simulink model "referee"  (R2018a)
settings: Solver=VariableStepAuto  StartTime=0.0  StopTime=20  FixedStep=0.01  RelTol=1e-3
libraries: simulink x16, instrumentlib x2
settings Model: EnablePacing=on  Creator=U500304  LastModifiedBy=Rafael
settings SolverCC: ZeroCrossAlgorithm=Adaptive
settings DataIOCC: SaveOutput=off  SaveTime=off
settings DebuggingCC: MaxConsecutiveZCsMsg=none

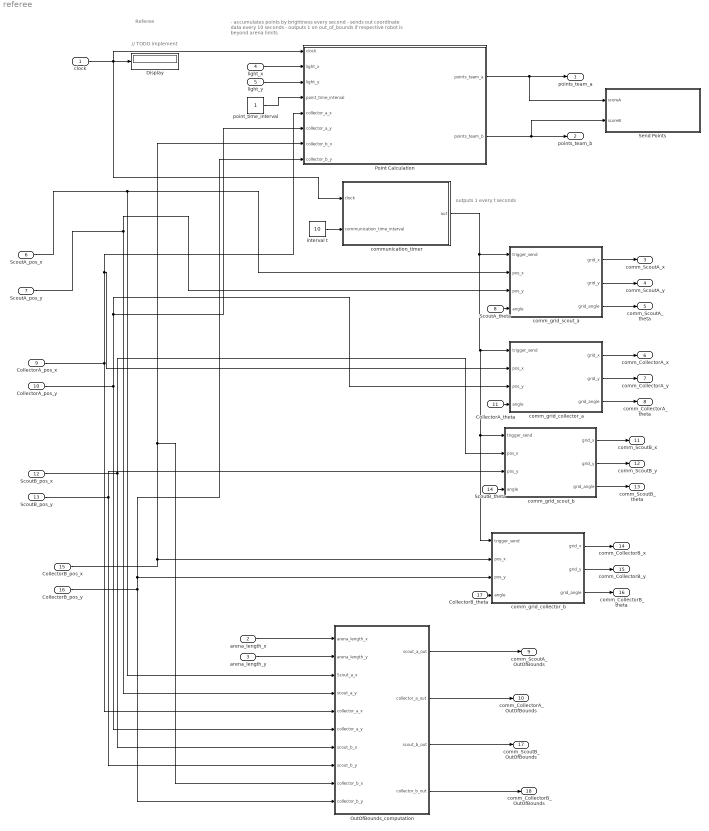
== system referee ==
  note: - accumulates points by brightness every second
      | - sends out coordinate data every 10 seconds
      | - outputs 1 on out_of_bounds if respective robot is beyond arena limits
  note: outputs 1 every t seconds
  note: // TODO implement
  note: Referee
  clock : Inport  OutDataTypeStr=double  PortDimensions=1  SampleTime=0
  arena_length_x : Inport  Port=2
  arena_length_y : Inport  Port=3
  light_x : Inport  Port=4
  light_y : Inport  Port=5
  ScoutA_pos_x : Inport  Port=6
  ScoutA_pos_y : Inport  Port=7
  ScoutA_theta : Inport  Port=8
  CollectorA_pos_x : Inport  Port=9
  CollectorA_pos_y : Inport  Port=10
  CollectorA_theta : Inport  Port=11
  ScoutB_pos_x : Inport  Port=12
  ScoutB_pos_y : Inport  Port=13
  ScoutB_theta : Inport  Port=14
  CollectorB_pos_x : Inport  Port=15
  CollectorB_pos_y : Inport  Port=16
  CollectorB_theta : Inport  Port=17
  Display : Display
  OutOfBounds_computation : Subsystem
  Point Calculation : Subsystem
  Send Points : Subsystem
  comm_grid_collector_a : Subsystem
  comm_grid_collector_b : Subsystem
  "comm_grid_scout_a " : Subsystem
  comm_grid_scout_b : Subsystem
  communication_timer : Subsystem
  interval t : Constant  Value=10
  point_time_interval : Constant
  points_team_a : Outport
  points_team_b : Outport  Port=2
  comm_ScoutA_x : Outport  Port=3
  comm_ScoutA_y : Outport  Port=4
  comm_ScoutA_theta : Outport  Port=5
  comm_CollectorA_x : Outport  Port=6
  comm_CollectorA_y : Outport  Port=7
  comm_CollectorA_theta : Outport  Port=8
  comm_ScoutA_OutOfBounds : Outport  Port=9
  comm_CollectorA_OutOfBounds : Outport  Port=10
  comm_ScoutB_x : Outport  Port=11
  comm_ScoutB_y : Outport  Port=12
  comm_ScoutB_theta : Outport  Port=13
  comm_CollectorB_x : Outport  Port=14
  comm_CollectorB_y : Outport  Port=15
  comm_CollectorB_theta : Outport  Port=16
  comm_ScoutB_OutOfBounds : Outport  Port=17
  comm_CollectorB_OutOfBounds : Outport  Port=18
  wires:
  arena_length_x/1 -> OutOfBounds_computation/1(arena_length_x)
  arena_length_y/1 -> OutOfBounds_computation/2(arena_length_y)
  ScoutA_pos_x/1 -> "comm_grid_scout_a "/2(pos_x), OutOfBounds_computation/3(Scout_a_x)
  ScoutA_pos_y/1 -> "comm_grid_scout_a "/3(pos_y), OutOfBounds_computation/4(scout_a_y)
  CollectorA_pos_x/1 -> comm_grid_collector_a/2(pos_x), Point Calculation/5(collector_a_x), OutOfBounds_computation/5(collector_a_x)
  CollectorA_pos_y/1 -> comm_grid_collector_a/3(pos_y), Point Calculation/6(collector_a_y), OutOfBounds_computation/6(collector_a_y)
  ScoutB_pos_x/1 -> comm_grid_scout_b/2(pos_x), OutOfBounds_computation/7(scout_b_x)
  ScoutB_pos_y/1 -> comm_grid_scout_b/3(pos_y), OutOfBounds_computation/8(scout_b_y)
  CollectorB_pos_x/1 -> Point Calculation/7(collector_b_x), OutOfBounds_computation/9(collector_b_x), comm_grid_collector_b/2(pos_x)
  CollectorB_pos_y/1 -> Point Calculation/8(collector_b_y), comm_grid_collector_b/3(pos_y), OutOfBounds_computation/10(collector_b_y)
  OutOfBounds_computation/1(scout_a_out) -> comm_ScoutA_OutOfBounds/1
  OutOfBounds_computation/2(collector_a_out) -> comm_CollectorA_OutOfBounds/1
  OutOfBounds_computation/3(scout_b_out) -> comm_ScoutB_OutOfBounds/1
  OutOfBounds_computation/4(collector_b_out) -> comm_CollectorB_OutOfBounds/1
  light_x/1 -> Point Calculation/2(light_x)
  light_y/1 -> Point Calculation/3(light_y)
  point_time_interval/1 -> Point Calculation/4(point_time_interval)
  Point Calculation/1(points_team_a) -> Send Points/1(scoreA), points_team_a/1
  Point Calculation/2(points_team_b) -> points_team_b/1, Send Points/2(scoreB)
  clock/1 -> communication_timer/1(clock), Point Calculation/1("clock "), Display/1
  interval t/1 -> communication_timer/2(communication_time_interval)
  communication_timer/1(out) -> comm_grid_collector_b/1(trigger_send), comm_grid_scout_b/1(trigger_send), comm_grid_collector_a/1(trigger_send), "comm_grid_scout_a "/1(trigger_send)
  ScoutA_theta/1 -> "comm_grid_scout_a "/4(angle)
  "comm_grid_scout_a "/1(grid_x) -> comm_ScoutA_x/1
  "comm_grid_scout_a "/2(grid_y) -> comm_ScoutA_y/1
  "comm_grid_scout_a "/3(grid_angle) -> comm_ScoutA_theta/1
  CollectorA_theta/1 -> comm_grid_collector_a/4(angle)
  comm_grid_collector_a/1(grid_x) -> comm_CollectorA_x/1
  comm_grid_collector_a/2(grid_y) -> comm_CollectorA_y/1
  comm_grid_collector_a/3(grid_angle) -> comm_CollectorA_theta/1
  ScoutB_theta/1 -> comm_grid_scout_b/4(angle)
  comm_grid_scout_b/1(grid_x) -> comm_ScoutB_x/1
  comm_grid_scout_b/2(grid_y) -> comm_ScoutB_y/1
  comm_grid_scout_b/3(grid_angle) -> comm_ScoutB_theta/1
  CollectorB_theta/1 -> comm_grid_collector_b/4(angle)
  comm_grid_collector_b/1(grid_x) -> comm_CollectorB_x/1
  comm_grid_collector_b/2(grid_y) -> comm_CollectorB_y/1
  comm_grid_collector_b/3(grid_angle) -> comm_CollectorB_theta/1

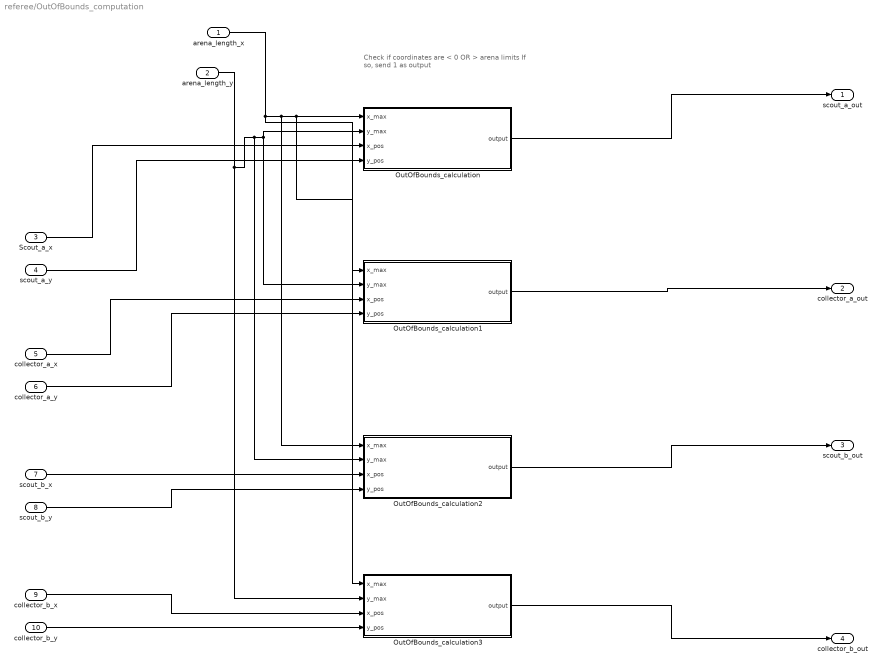
== system referee/OutOfBounds_computation ==
  note: Check if coordinates are < 0 OR > arena limits
      | If so, send 1 as output
  arena_length_x : Inport
  arena_length_y : Inport  Port=2
  Scout_a_x : Inport  Port=3
  scout_a_y : Inport  Port=4
  collector_a_x : Inport  Port=5
  collector_a_y : Inport  Port=6
  scout_b_x : Inport  Port=7
  scout_b_y : Inport  Port=8
  collector_b_x : Inport  Port=9
  collector_b_y : Inport  Port=10
  OutOfBounds_calculation : Subsystem
  OutOfBounds_calculation1 : Subsystem
  OutOfBounds_calculation2 : Subsystem
  OutOfBounds_calculation3 : Subsystem
  scout_a_out : Outport
  collector_a_out : Outport  Port=2
  scout_b_out : Outport  Port=3
  collector_b_out : Outport  Port=4
  wires:
  OutOfBounds_calculation/1(output) -> scout_a_out/1
  arena_length_x/1 -> OutOfBounds_calculation3/1(x_max), OutOfBounds_calculation2/1(x_max), OutOfBounds_calculation1/1(x_max), OutOfBounds_calculation/1(x_max)
  arena_length_y/1 -> OutOfBounds_calculation3/2(y_max), OutOfBounds_calculation2/2(y_max), OutOfBounds_calculation/2(y_max), OutOfBounds_calculation1/2(y_max)
  collector_b_y/1 -> OutOfBounds_calculation3/4(y_pos)
  OutOfBounds_calculation1/1(output) -> collector_a_out/1
  collector_b_x/1 -> OutOfBounds_calculation3/3(x_pos)
  collector_a_y/1 -> OutOfBounds_calculation1/4(y_pos)
  scout_b_x/1 -> OutOfBounds_calculation2/3(x_pos)
  OutOfBounds_calculation2/1(output) -> scout_b_out/1
  Scout_a_x/1 -> OutOfBounds_calculation/3(x_pos)
  scout_a_y/1 -> OutOfBounds_calculation/4(y_pos)
  OutOfBounds_calculation3/1(output) -> collector_b_out/1
  scout_b_y/1 -> OutOfBounds_calculation2/4(y_pos)
  collector_a_x/1 -> OutOfBounds_calculation1/3(x_pos)

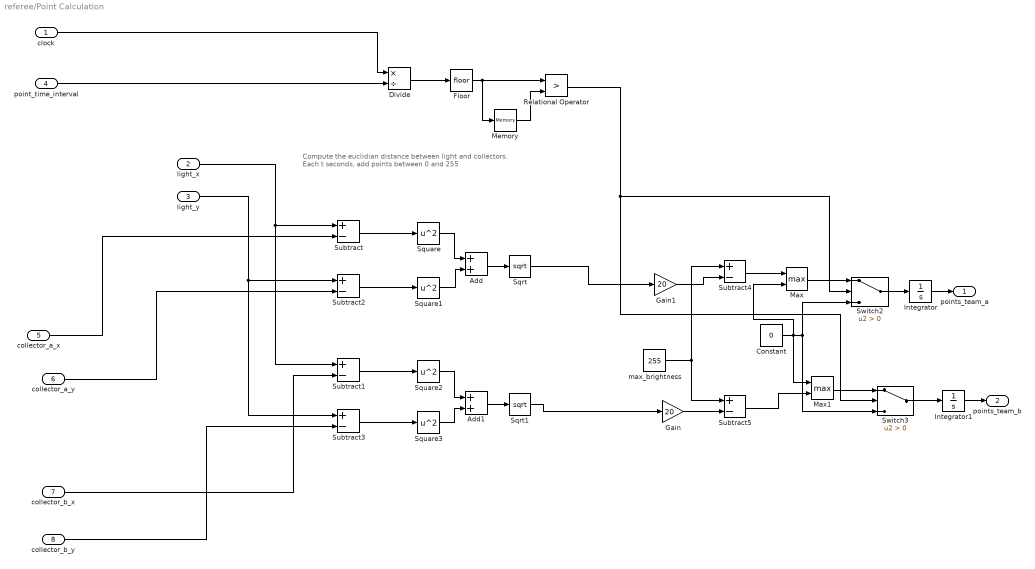
== system referee/Point Calculation ==
  note: Compute the euclidian distance between light and collectors.
      | Each t seconds, add points between 0 and 255
  "clock " : Inport
  light_x : Inport  Port=2
  light_y : Inport  Port=3
  point_time_interval : Inport  Port=4
  collector_a_x : Inport  Port=5
  collector_a_y : Inport  Port=6
  collector_b_x : Inport  Port=7
  collector_b_y : Inport  Port=8
  Add : Sum
  Add1 : Sum
  Constant : Constant  Value=0
  Divide : Product  Inputs=*/
  Floor : Rounding
  Gain : Gain  Gain=20
  Gain1 : Gain  Gain=20
  Integrator : Integrator
  Integrator1 : Integrator
  Max : MinMax  Function=max  Inputs=2
  Max1 : MinMax  Function=max  Inputs=2
  Memory : Memory
  Relational Operator : RelationalOperator  Operator=>  OutDataTypeStr=boolean  RndMeth=Simplest
  Sqrt : Sqrt  SaturateOnIntegerOverflow=on
  Sqrt1 : Sqrt  SaturateOnIntegerOverflow=on
  Square{,1..3} (4 alike) : Math  Operator=square  SaturateOnIntegerOverflow=on
  Subtract{,1..5} (6 alike) : Sum  Inputs=+-
  Switch2 : Switch  Criteria=u2 > Threshold
  Switch3 : Switch  Criteria=u2 > Threshold
  max_brightness : Constant  Value=255
  points_team_a : Outport
  points_team_b : Outport  Port=2
  wires:
  Divide/1 -> Floor/1
  light_y/1 -> Subtract3/1, Subtract2/1
  Memory/1 -> Relational Operator/2
  light_x/1 -> Subtract1/1, Subtract/1
  Square/1 -> Add/1
  Floor/1 -> Relational Operator/1, Memory/1
  collector_b_y/1 -> Subtract3/2
  Add/1 -> Sqrt/1
  Constant/1 -> Max1/1, Max/2, Switch3/3, Switch2/3
  Relational Operator/1 -> Switch3/2, Switch2/2
  point_time_interval/1 -> Divide/2
  collector_a_x/1 -> Subtract/2
  Square3/1 -> Add1/2
  Subtract2/1 -> Square1/1
  Subtract/1 -> Square/1
  Subtract1/1 -> Square2/1
  Add1/1 -> Sqrt1/1
  Square2/1 -> Add1/1
  Subtract3/1 -> Square3/1
  Square1/1 -> Add/2
  collector_a_y/1 -> Subtract2/2
  collector_b_x/1 -> Subtract1/2
  "clock "/1 -> Divide/1
  max_brightness/1 -> Subtract5/1, Subtract4/1
  Sqrt/1 -> Gain1/1
  Gain1/1 -> Subtract4/2
  Subtract4/1 -> Max/1
  Sqrt1/1 -> Gain/1
  Gain/1 -> Subtract5/2
  Subtract5/1 -> Max1/2
  Max/1 -> Switch2/1
  Max1/1 -> Switch3/1
  Integrator/1 -> points_team_a/1
  Integrator1/1 -> points_team_b/1
  Switch3/1 -> Integrator1/1
  Switch2/1 -> Integrator/1

== system referee/Send Points ==
  scoreA : Inport
  scoreB : Inport  Port=2
  Rate Transition5 : RateTransition  OutPortSampleTime=0.1
  Rate Transition6 : RateTransition  OutPortSampleTime=0.1
  tcp_send_scoreA : instrumentlib/TCP//IP Send  Host=localhost  Port=50015  EnableBlockingMode=on  Timeout=1  ByteOrder=LittleEndian  TransferDelay=on
      settings: SourceProductName=Instrument Control Toolbox
  tcp_send_scoreB : instrumentlib/TCP//IP Send  Host=localhost  Port=50016  EnableBlockingMode=on  Timeout=1  ByteOrder=LittleEndian  TransferDelay=on
      settings: SourceProductName=Instrument Control Toolbox
  wires:
  scoreA/1 -> Rate Transition5/1
  scoreB/1 -> Rate Transition6/1
  Rate Transition5/1 -> tcp_send_scoreA/1
  Rate Transition6/1 -> tcp_send_scoreB/1

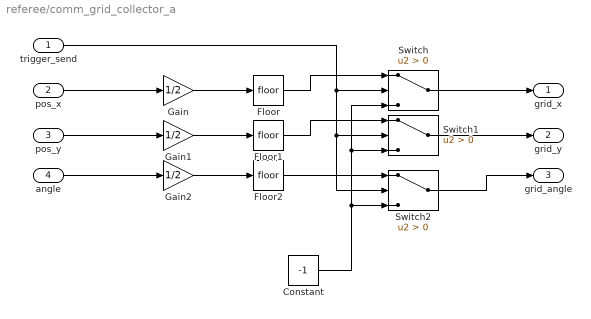
== system referee/comm_grid_collector_a ==
  trigger_send : Inport
  pos_x : Inport  Port=2
  pos_y : Inport  Port=3
  angle : Inport  Port=4
  Constant : Constant  Value=-1
  Floor : Rounding
  Floor1 : Rounding
  Floor2 : Rounding
  Gain : Gain  Gain=1/2
  Gain1 : Gain  Gain=1/2
  Gain2 : Gain  Gain=1/2
  Switch : Switch  Criteria=u2 > Threshold
  Switch1 : Switch  Criteria=u2 > Threshold
  Switch2 : Switch  Criteria=u2 > Threshold
  grid_x : Outport
  grid_y : Outport  Port=2
  grid_angle : Outport  Port=3
  wires:
  Switch2/1 -> grid_angle/1
  Floor/1 -> Switch/1
  Switch/1 -> grid_x/1
  Switch1/1 -> grid_y/1
  angle/1 -> Gain2/1
  Gain2/1 -> Floor2/1
  Floor1/1 -> Switch1/1
  pos_x/1 -> Gain/1
  Gain/1 -> Floor/1
  Gain1/1 -> Floor1/1
  pos_y/1 -> Gain1/1
  trigger_send/1 -> Switch/2, Switch2/2, Switch1/2
  Constant/1 -> Switch1/3, Switch/3, Switch2/3
  Floor2/1 -> Switch2/1

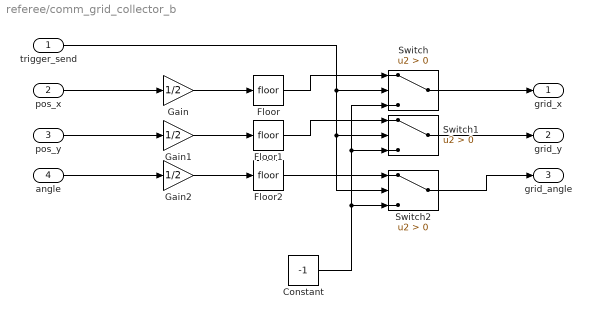
== system referee/comm_grid_collector_b ==
  trigger_send : Inport
  pos_x : Inport  Port=2
  pos_y : Inport  Port=3
  angle : Inport  Port=4
  Constant : Constant  Value=-1
  Floor : Rounding
  Floor1 : Rounding
  Floor2 : Rounding
  Gain : Gain  Gain=1/2
  Gain1 : Gain  Gain=1/2
  Gain2 : Gain  Gain=1/2
  Switch : Switch  Criteria=u2 > Threshold
  Switch1 : Switch  Criteria=u2 > Threshold
  Switch2 : Switch  Criteria=u2 > Threshold
  grid_x : Outport
  grid_y : Outport  Port=2
  grid_angle : Outport  Port=3
  wires:
  Floor2/1 -> Switch2/1
  Constant/1 -> Switch2/3, Switch/3, Switch1/3
  trigger_send/1 -> Switch1/2, Switch2/2, Switch/2
  pos_y/1 -> Gain1/1
  Gain1/1 -> Floor1/1
  Gain/1 -> Floor/1
  pos_x/1 -> Gain/1
  Floor1/1 -> Switch1/1
  Gain2/1 -> Floor2/1
  angle/1 -> Gain2/1
  Switch1/1 -> grid_y/1
  Switch/1 -> grid_x/1
  Floor/1 -> Switch/1
  Switch2/1 -> grid_angle/1

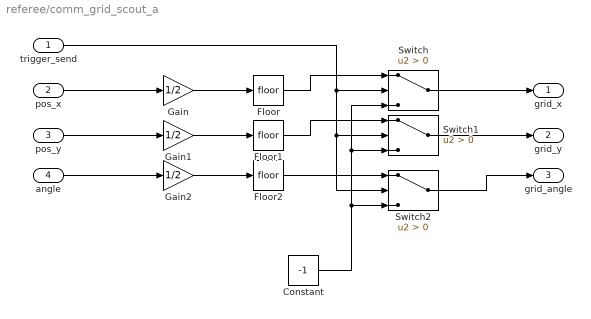
== system referee/comm_grid_scout_a  ==
  trigger_send : Inport
  pos_x : Inport  Port=2
  pos_y : Inport  Port=3
  angle : Inport  Port=4
  Constant : Constant  Value=-1
  Floor : Rounding
  Floor1 : Rounding
  Floor2 : Rounding
  Gain : Gain  Gain=1/2
  Gain1 : Gain  Gain=1/2
  Gain2 : Gain  Gain=1/2
  Switch : Switch  Criteria=u2 > Threshold
  Switch1 : Switch  Criteria=u2 > Threshold
  Switch2 : Switch  Criteria=u2 > Threshold
  grid_x : Outport
  grid_y : Outport  Port=2
  grid_angle : Outport  Port=3
  wires:
  Floor2/1 -> Switch2/1
  Constant/1 -> Switch2/3, Switch/3, Switch1/3
  trigger_send/1 -> Switch1/2, Switch2/2, Switch/2
  pos_y/1 -> Gain1/1
  Gain1/1 -> Floor1/1
  Gain/1 -> Floor/1
  pos_x/1 -> Gain/1
  Floor1/1 -> Switch1/1
  Gain2/1 -> Floor2/1
  angle/1 -> Gain2/1
  Switch1/1 -> grid_y/1
  Switch/1 -> grid_x/1
  Floor/1 -> Switch/1
  Switch2/1 -> grid_angle/1

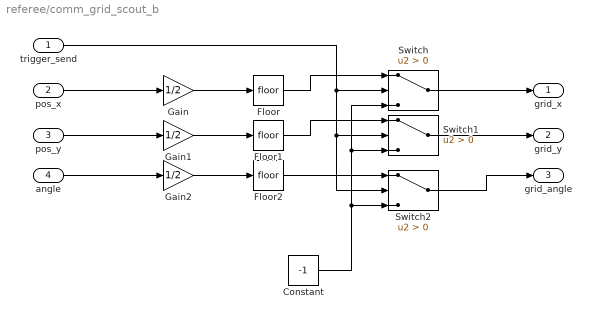
== system referee/comm_grid_scout_b ==
  trigger_send : Inport
  pos_x : Inport  Port=2
  pos_y : Inport  Port=3
  angle : Inport  Port=4
  Constant : Constant  Value=-1
  Floor : Rounding
  Floor1 : Rounding
  Floor2 : Rounding
  Gain : Gain  Gain=1/2
  Gain1 : Gain  Gain=1/2
  Gain2 : Gain  Gain=1/2
  Switch : Switch  Criteria=u2 > Threshold
  Switch1 : Switch  Criteria=u2 > Threshold
  Switch2 : Switch  Criteria=u2 > Threshold
  grid_x : Outport
  grid_y : Outport  Port=2
  grid_angle : Outport  Port=3
  wires:
  Switch2/1 -> grid_angle/1
  Floor/1 -> Switch/1
  Switch/1 -> grid_x/1
  Switch1/1 -> grid_y/1
  angle/1 -> Gain2/1
  Gain2/1 -> Floor2/1
  Floor1/1 -> Switch1/1
  pos_x/1 -> Gain/1
  Gain/1 -> Floor/1
  Gain1/1 -> Floor1/1
  pos_y/1 -> Gain1/1
  trigger_send/1 -> Switch/2, Switch2/2, Switch1/2
  Constant/1 -> Switch1/3, Switch/3, Switch2/3
  Floor2/1 -> Switch2/1

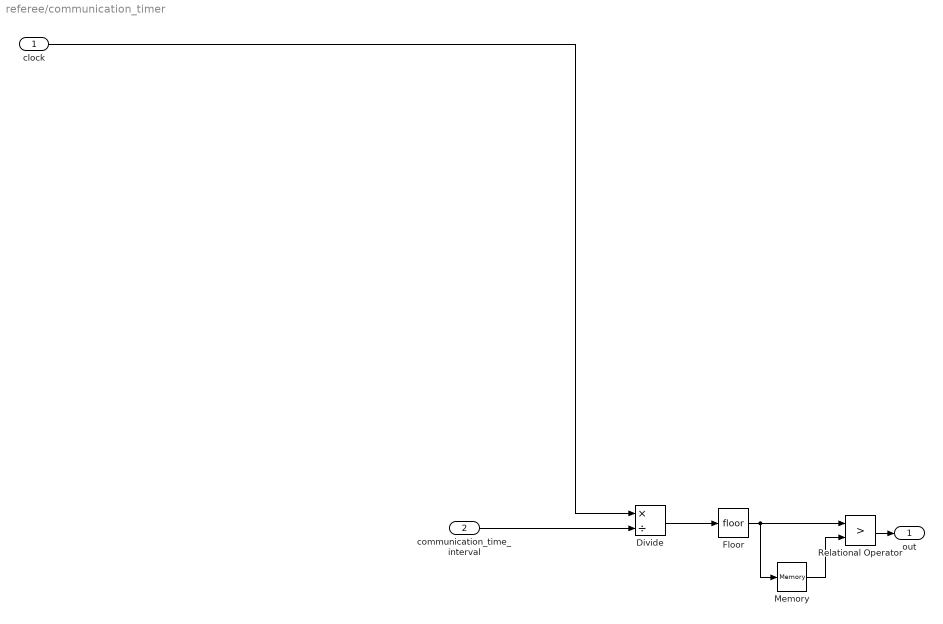
== system referee/communication_timer ==
  clock : Inport
  communication_time_interval : Inport  Port=2
  Divide : Product  Inputs=*/
  Floor : Rounding
  Memory : Memory
  Relational Operator : RelationalOperator  Operator=>  OutDataTypeStr=boolean  RndMeth=Simplest
  out : Outport
  wires:
  Divide/1 -> Floor/1
  Memory/1 -> Relational Operator/2
  Floor/1 -> Relational Operator/1, Memory/1
  communication_time_interval/1 -> Divide/2
  clock/1 -> Divide/1
  Relational Operator/1 -> out/1

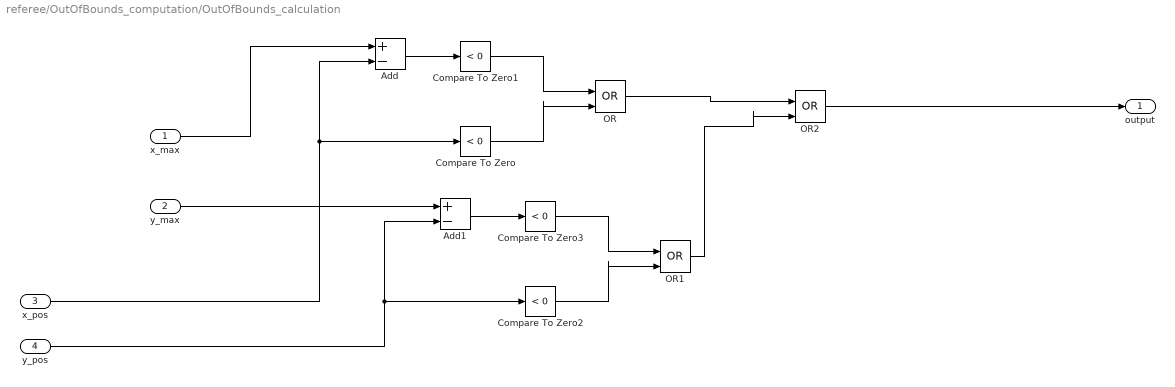
== system referee/OutOfBounds_computation/OutOfBounds_calculation ==
  x_max : Inport
  y_max : Inport  Port=2
  x_pos : Inport  Port=3
  y_pos : Inport  Port=4
  Add : Sum  Inputs=+-
  Add1 : Sum  Inputs=+-
  Compare To Zero{,1..3} (4 alike) : simulink/Logic and Bit Operations/Compare To Zero  relop=<  OutDataTypeStr=boolean
  OR : Logic  Operator=OR  IconShape=distinctive  AllPortsSameDT=off  OutDataTypeStr=boolean
  OR1 : Logic  Operator=OR  IconShape=distinctive  AllPortsSameDT=off  OutDataTypeStr=boolean
  OR2 : Logic  Operator=OR  IconShape=distinctive  AllPortsSameDT=off  OutDataTypeStr=boolean
  output : Outport
  wires:
  Add1/1 -> Compare To Zero3/1
  Compare To Zero3/1 -> OR1/1
  x_pos/1 -> Add/2, Compare To Zero/1
  x_max/1 -> Add/1
  OR/1 -> OR2/1
  y_pos/1 -> Add1/2, Compare To Zero2/1
  Compare To Zero2/1 -> OR1/2
  Compare To Zero/1 -> OR/2
  OR1/1 -> OR2/2
  Add/1 -> Compare To Zero1/1
  Compare To Zero1/1 -> OR/1
  y_max/1 -> Add1/1
  OR2/1 -> output/1

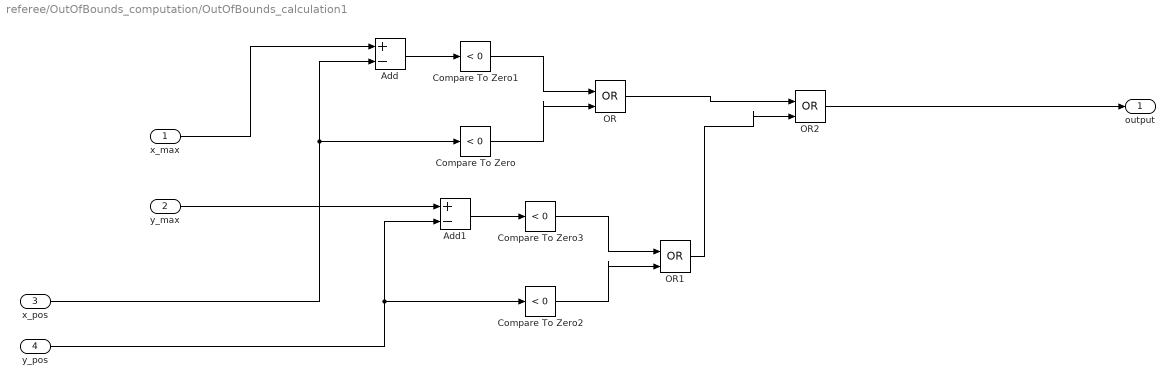
== system referee/OutOfBounds_computation/OutOfBounds_calculation1 ==
  x_max : Inport
  y_max : Inport  Port=2
  x_pos : Inport  Port=3
  y_pos : Inport  Port=4
  Add : Sum  Inputs=+-
  Add1 : Sum  Inputs=+-
  Compare To Zero{,1..3} (4 alike) : simulink/Logic and Bit Operations/Compare To Zero  relop=<  OutDataTypeStr=boolean
  OR : Logic  Operator=OR  IconShape=distinctive  AllPortsSameDT=off  OutDataTypeStr=boolean
  OR1 : Logic  Operator=OR  IconShape=distinctive  AllPortsSameDT=off  OutDataTypeStr=boolean
  OR2 : Logic  Operator=OR  IconShape=distinctive  AllPortsSameDT=off  OutDataTypeStr=boolean
  output : Outport
  wires:
  OR2/1 -> output/1
  y_max/1 -> Add1/1
  Compare To Zero1/1 -> OR/1
  Add/1 -> Compare To Zero1/1
  OR1/1 -> OR2/2
  Compare To Zero/1 -> OR/2
  Compare To Zero2/1 -> OR1/2
  y_pos/1 -> Compare To Zero2/1, Add1/2
  OR/1 -> OR2/1
  x_max/1 -> Add/1
  x_pos/1 -> Compare To Zero/1, Add/2
  Compare To Zero3/1 -> OR1/1
  Add1/1 -> Compare To Zero3/1

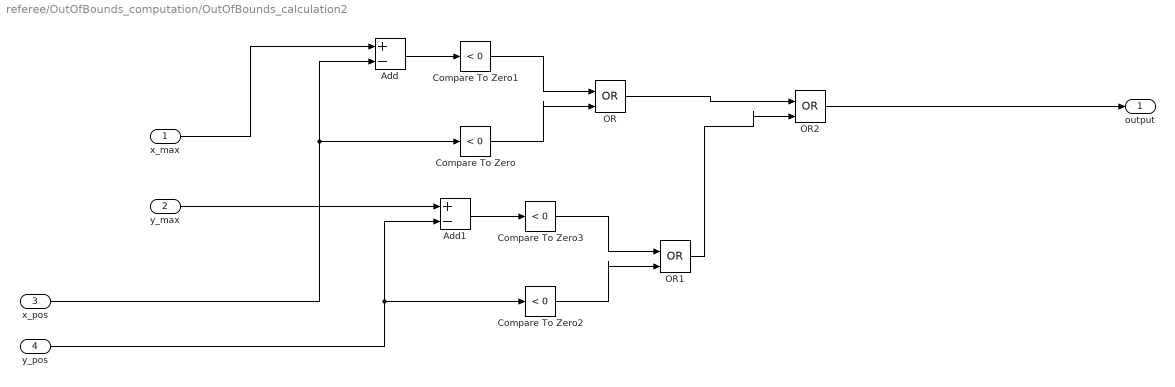
== system referee/OutOfBounds_computation/OutOfBounds_calculation2 ==
  x_max : Inport
  y_max : Inport  Port=2
  x_pos : Inport  Port=3
  y_pos : Inport  Port=4
  Add : Sum  Inputs=+-
  Add1 : Sum  Inputs=+-
  Compare To Zero{,1..3} (4 alike) : simulink/Logic and Bit Operations/Compare To Zero  relop=<  OutDataTypeStr=boolean
  OR : Logic  Operator=OR  IconShape=distinctive  AllPortsSameDT=off  OutDataTypeStr=boolean
  OR1 : Logic  Operator=OR  IconShape=distinctive  AllPortsSameDT=off  OutDataTypeStr=boolean
  OR2 : Logic  Operator=OR  IconShape=distinctive  AllPortsSameDT=off  OutDataTypeStr=boolean
  output : Outport
  wires:
  Add1/1 -> Compare To Zero3/1
  Compare To Zero3/1 -> OR1/1
  x_pos/1 -> Add/2, Compare To Zero/1
  x_max/1 -> Add/1
  OR/1 -> OR2/1
  y_pos/1 -> Add1/2, Compare To Zero2/1
  Compare To Zero2/1 -> OR1/2
  Compare To Zero/1 -> OR/2
  OR1/1 -> OR2/2
  Add/1 -> Compare To Zero1/1
  Compare To Zero1/1 -> OR/1
  y_max/1 -> Add1/1
  OR2/1 -> output/1

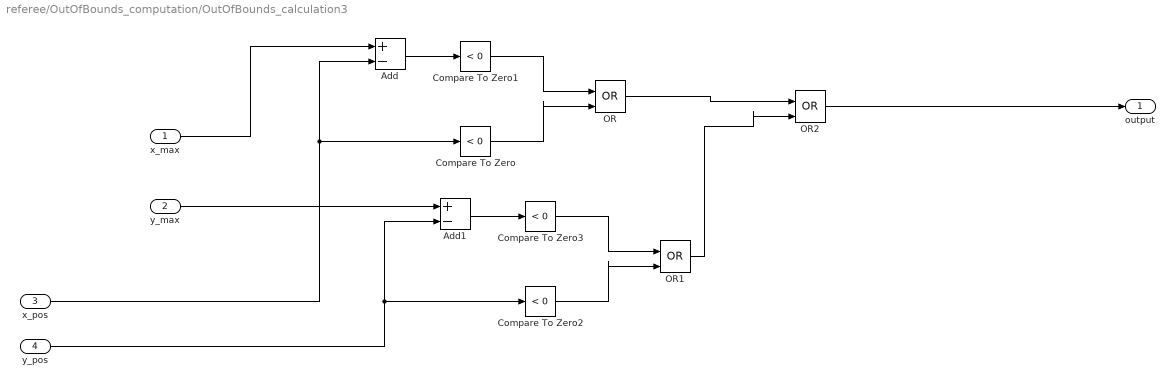
== system referee/OutOfBounds_computation/OutOfBounds_calculation3 ==
  x_max : Inport
  y_max : Inport  Port=2
  x_pos : Inport  Port=3
  y_pos : Inport  Port=4
  Add : Sum  Inputs=+-
  Add1 : Sum  Inputs=+-
  Compare To Zero{,1..3} (4 alike) : simulink/Logic and Bit Operations/Compare To Zero  relop=<  OutDataTypeStr=boolean
  OR : Logic  Operator=OR  IconShape=distinctive  AllPortsSameDT=off  OutDataTypeStr=boolean
  OR1 : Logic  Operator=OR  IconShape=distinctive  AllPortsSameDT=off  OutDataTypeStr=boolean
  OR2 : Logic  Operator=OR  IconShape=distinctive  AllPortsSameDT=off  OutDataTypeStr=boolean
  output : Outport
  wires:
  OR2/1 -> output/1
  y_max/1 -> Add1/1
  Compare To Zero1/1 -> OR/1
  Add/1 -> Compare To Zero1/1
  OR1/1 -> OR2/2
  Compare To Zero/1 -> OR/2
  Compare To Zero2/1 -> OR1/2
  y_pos/1 -> Compare To Zero2/1, Add1/2
  OR/1 -> OR2/1
  x_max/1 -> Add/1
  x_pos/1 -> Compare To Zero/1, Add/2
  Compare To Zero3/1 -> OR1/1
  Add1/1 -> Compare To Zero3/1
